simulink model "nlMiP_HW4"  (R2019b)
settings: Solver=VariableStepAuto  StartTime=0.0  StopTime=10.0  RelTol=1e-3
values from neighbouring files (symbols this model uses):
  a = 2*I_w+(m_b+2*m_w)*r^2    (= 0.0004887601928)    [ZhuoMiPparameters.m]    (also in myEig.m)
  b = m_b*r*l    (= 0.000321912)    [ZhuoMiPparameters.m]    (also in myEig.m)
  c = I_b+m_b*l^2    (= 0.000740848)    [ZhuoMiPparameters.m]    (also in myEig.m)
  d = m_b*g*l    (= 0.0927864)    [ZhuoMiPparameters.m]    (also in mathieu_equation.m = [x(2);-(alpha+beta*cos(t)*x(1))]; myEig.m)
  e = 2*G_r*s/V_max    (= 0.0288405405405)    [ZhuoMiPparameters.m]    (also in myEig.m)
  j = 2*G_r^2*k    (= 0.00431326670455)    [ZhuoMiPparameters.m]    (also in myEig.m)
undefined symbols (not defined in the file or in its folder): ALCBKDmIp, DLDmIp, KLDmIp, LLDmIp
libraries: simulink x2
settings Model: Creator=bob  LastModifiedBy=leoli

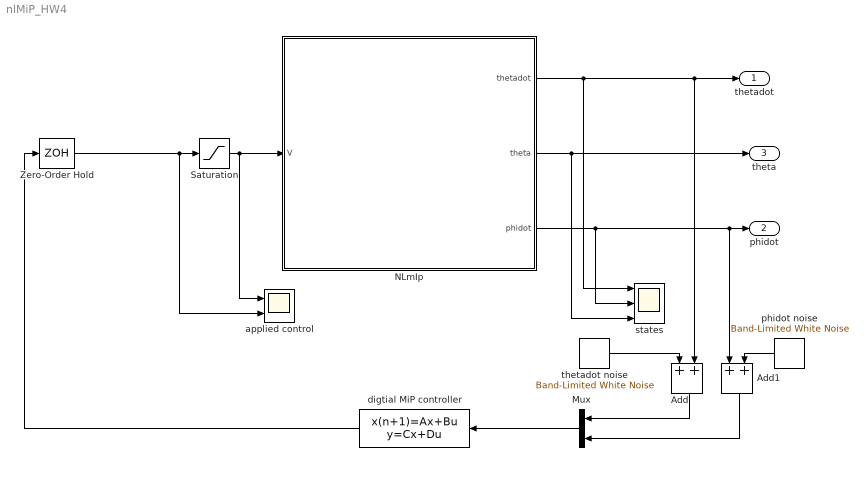
== system nlMiP_HW4 ==
  Add : Sum
  Add1 : Sum  Inputs=2
  Mux : Mux  Inputs=2
  NLmIp : Subsystem
  Saturation : Saturate  UpperLimit=6  LowerLimit=-6
  Zero-Order Hold : ZeroOrderHold  SampleTime=.01
  applied control : Scope  NumInputPorts=2
  digtial MiP controller : DiscreteStateSpace  A=ALCBKDmIp  B=LLDmIp  C=KLDmIp  D=DLDmIp  SampleTime=0.01
  phidot noise : simulink/Sources/Band-Limited White Noise  Cov=0  Ts=.01  seed=[23341]
  states : Scope  NumInputPorts=3
  thetadot noise : simulink/Sources/Band-Limited White Noise  Cov=0  Ts=0.01  seed=[23341]
  thetadot : Outport
  phidot : Outport  Port=2
  theta : Outport  Port=3
  wires:
  NLmIp/1(thetadot) -> states/1, Add/2, thetadot/1
  NLmIp/2(theta) -> states/3, theta/1
  NLmIp/3(phidot) -> states/2, Add1/1, phidot/1
  Saturation/1 -> NLmIp/1(V), applied control/1
  Zero-Order Hold/1 -> applied control/2, Saturation/1
  Mux/1 -> digtial MiP controller/1
  digtial MiP controller/1 -> Zero-Order Hold/1
  thetadot noise/1 -> Add/1
  phidot noise/1 -> Add1/2
  Add/1 -> Mux/1
  Add1/1 -> Mux/2

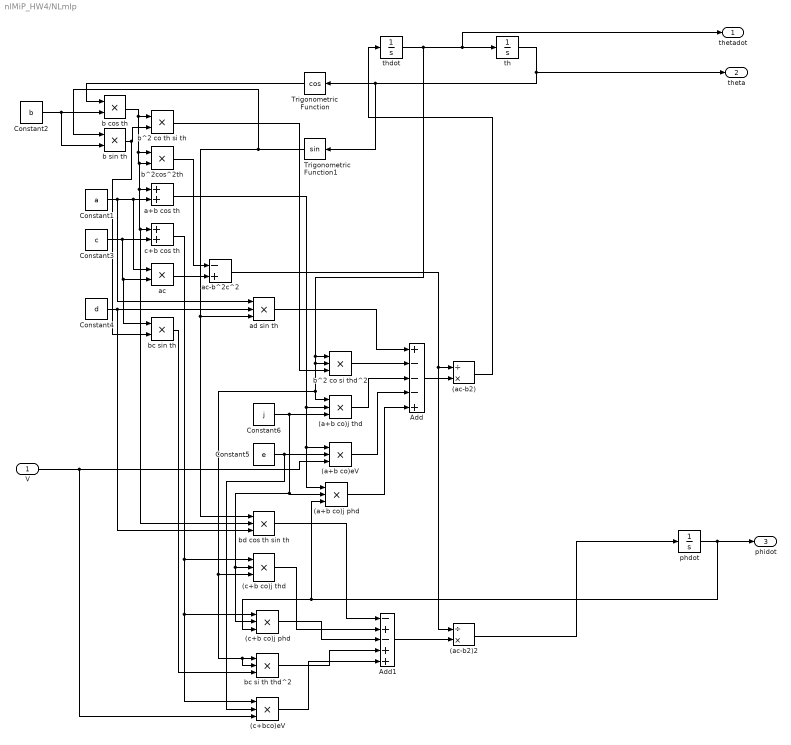
== system nlMiP_HW4/NLmIp ==
  V : Inport
  (a+b co)eV : Product  Inputs=3
  (a+b co)j phd : Product  Inputs=3
  (a+b co)j thd : Product  Inputs=3
  (ac-b2) : Product  Inputs=/*
  (ac-b2)2 : Product  Inputs=/*
  (c+b co)j phd : Product  Inputs=3
  (c+b co)j thd : Product  Inputs=3
  (c+bco)eV : Product  Inputs=3
  Add : Sum  Inputs=+---+
  Add1 : Sum  Inputs=-+-++
  Constant1 : Constant  Value=a
  Constant2 : Constant  Value=b
  Constant3 : Constant  Value=c
  Constant4 : Constant  Value=d
  Constant5 : Constant  Value=e
  Constant6 : Constant  Value=j
  Trigonometric Function : Trigonometry  Operator=cos
  Trigonometric Function1 : Trigonometry
  a+b cos th : Sum
  ac : Product
  ac-b^2c^2 : Sum  Inputs=-+
  ad sin th : Product  Inputs=3
  b cos th : Product
  b sin th : Product
  b^2 co si thd^2 : Product  Inputs=3
  b^2 co th si th : Product
  b^2cos^2th : Product
  bc si th thd^2 : Product  Inputs=3
  bc sin th : Product
  bd cos th sin th : Product  Inputs=3
  c+b cos th : Sum
  phdot : Integrator
  th : Integrator  InitialCondition=0.06
  thdot : Integrator
  thetadot : Outport
  theta : Outport  Port=2
  phidot : Outport  Port=3
  wires:
  Trigonometric Function/1 -> b cos th/1
  (ac-b2)2/1 -> phdot/1
  V/1 -> (c+bco)eV/3, (a+b co)eV/3
  b^2 co th si th/1 -> b^2 co si thd^2/3
  ad sin th/1 -> Add/1
  c+b cos th/1 -> (c+bco)eV/1, (c+b co)j phd/1, (c+b co)j thd/1
  (c+b co)j phd/1 -> Add1/3
  Add/1 -> (ac-b2)/2
  (c+b co)j thd/1 -> Add1/2
  (a+b co)eV/1 -> Add/4
  b^2cos^2th/1 -> ac-b^2c^2/1
  b^2 co si thd^2/1 -> Add/2
  (ac-b2)/1 -> thdot/1
  (a+b co)j thd/1 -> Add/3
  b sin th/1 -> bc sin th/2, b^2 co th si th/2
  Constant5/1 -> (c+bco)eV/2, (a+b co)eV/2
  ac-b^2c^2/1 -> (ac-b2)2/1, (ac-b2)/1
  Constant3/1 -> bc sin th/1, ac/2, c+b cos th/2
  Constant6/1 -> (c+b co)j thd/2, (c+b co)j phd/2, (a+b co)j phd/2, (a+b co)j thd/3
  bd cos th sin th/1 -> Add1/1
  thdot/1 -> b^2 co si thd^2/1, b^2 co si thd^2/2, (c+b co)j thd/3, bc si th thd^2/2, bc si th thd^2/1, (a+b co)j thd/1, thetadot/1, th/1
  (a+b co)j phd/1 -> Add/5
  th/1 -> theta/1, Trigonometric Function1/1, Trigonometric Function/1
  Constant4/1 -> bd cos th sin th/3, ad sin th/2
  phdot/1 -> phidot/1, (c+b co)j phd/3, (a+b co)j phd/3
  Trigonometric Function1/1 -> b sin th/1, bd cos th sin th/1, ad sin th/3
  bc sin th/1 -> bc si th thd^2/3
  a+b cos th/1 -> (a+b co)j phd/1, (a+b co)eV/1, (a+b co)j thd/2
  Add1/1 -> (ac-b2)2/2
  ac/1 -> ac-b^2c^2/2
  bc si th thd^2/1 -> Add1/4
  (c+bco)eV/1 -> Add1/5
  b cos th/1 -> b^2 co th si th/1, bd cos th sin th/2, c+b cos th/1, a+b cos th/1, b^2cos^2th/2, b^2cos^2th/1
  Constant2/1 -> b sin th/2, b cos th/2
  Constant1/1 -> ad sin th/1, ac/1, a+b cos th/2
